simulink model "harness"  (R2021b)
settings: Solver=VariableStepAuto  StartTime=0.0  StopTime=inf  FixedStep=1/10  RelTol=1e-3
undefined symbols (not defined in the file): gaussian
libraries: simulink x2
settings Model: PacingRate=3  Creator=DAUIN-Win10  LastModifiedBy=maria

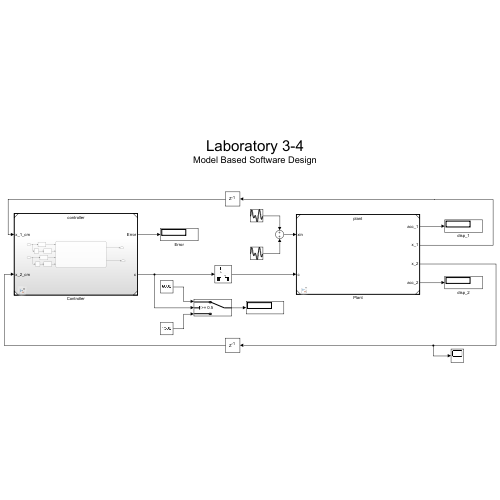
[thumbnail: Simulink's stored preview of the top-level diagram]
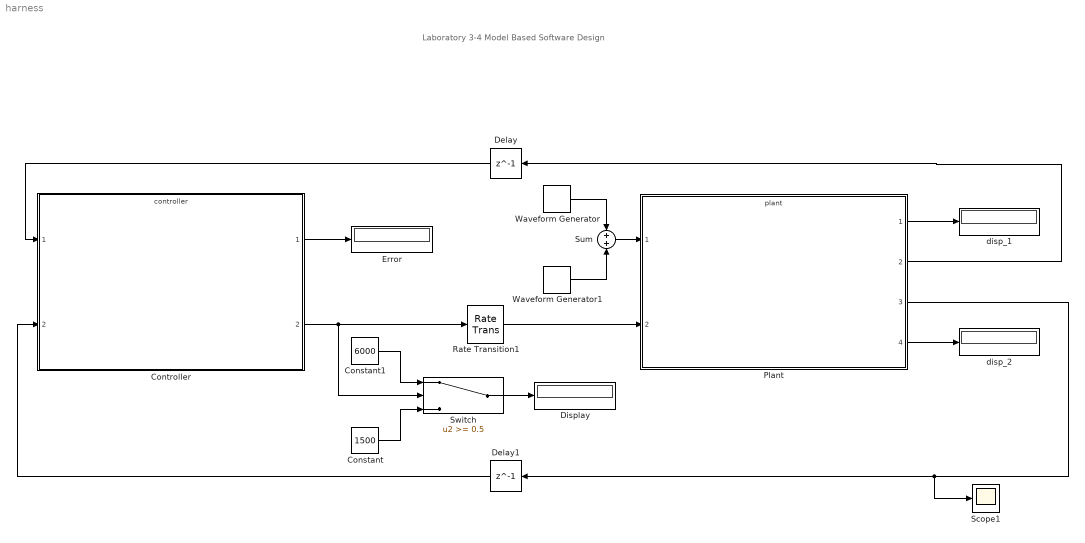
== system harness ==
  note: Laboratory 3-4
      | Model Based Software Design
  Constant : Constant  Value=1500
  Constant1 : Constant  Value=6000
  Controller : ModelReference  ModelNameDialog=controller  SimulationMode=Normal  ModelReferenceVersion=1.16
  Delay : Delay  DelayLength=1
  Delay1 : Delay  DelayLength=1
  Display : Display
  Error : Display
  Plant : ModelReference  ModelNameDialog=plant  SimulationMode=Normal  ModelReferenceVersion=1.14
  Rate Transition1 : RateTransition
  Scope1 : Scope
  Sum : Sum
  Switch : Switch  Threshold=0.5
  Waveform Generator : simulink/Sources/Waveform Generator  OutMin=[]  OutMax=[]  OutDataTypeStr=double  SelectedSignal=1  Signals=sin(0.2,1,0)  BlockNames=MultiportSwitch_b233b575e82d432  SampleTime=0.1
  Waveform Generator1 : simulink/Sources/Waveform Generator  OutMin=[]  OutMax=[]  OutDataTypeStr=double  SelectedSignal=1  Signals=gaussian(0,0.001,42)  BlockNames=MultiportSwitch_524d0bdf95c049e  SampleTime=0.1
  disp_1 : Display
  disp_2 : Display
  wires:
  Rate Transition1/1 -> Plant/2
  Delay1/1 -> Controller/2
  Plant/3 -> Scope1/1, Delay1/1
  Delay/1 -> Controller/1
  Controller/1 -> Error/1
  Plant/1 -> disp_1/1
  Waveform Generator1/1 -> Sum/2
  Waveform Generator/1 -> Sum/1
  Switch/1 -> Display/1
  Controller/2 -> Switch/2, Rate Transition1/1
  Sum/1 -> Plant/1
  Plant/4 -> disp_2/1
  Constant1/1 -> Switch/1
  Constant/1 -> Switch/3
  Plant/2 -> Delay/1
